simulink model "Schwingerkette_Model"  (R2014b)
settings: Solver=ode45  StartTime=0.0  StopTime=1  RelTol=1e-5
values from neighbouring files (symbols this model uses):
  c = 500    [Schwingerkette_Bearbeitungsfile.m]
  m = 0.5    [Schwingerkette_Bearbeitungsfile.m]
settings Model: Creator=edwardsue  LastModifiedBy=edwardsue

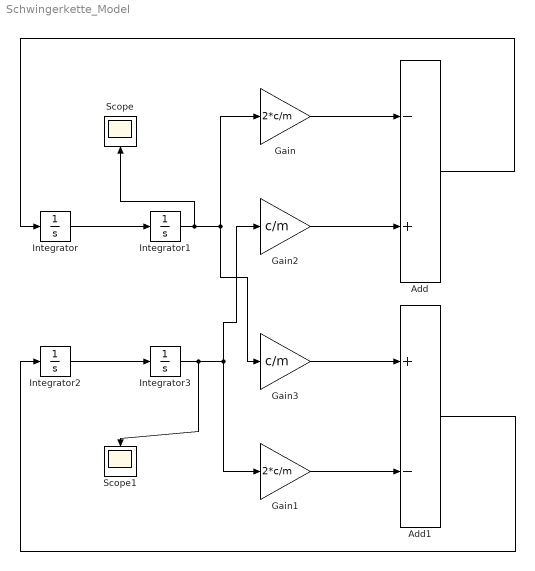
== system Schwingerkette_Model ==
  Add : Sum  Inputs=-+
  Add1 : Sum  Inputs=+-
  Gain : Gain  Gain=2*c/m
  Gain1 : Gain  Gain=2*c/m
  Gain2 : Gain  Gain=c/m
  Gain3 : Gain  Gain=c/m
  Integrator : Integrator
  Integrator1 : Integrator  InitialCondition=0.01
  Integrator2 : Integrator
  Integrator3 : Integrator  InitialCondition=0.01
  Scope : Scope
      settings: YMin=-1  YMax=1.5
  Scope1 : Scope
      settings: YMin=-1  YMax=1.5
  wires:
  Gain/1 -> Add/1
  Gain2/1 -> Add/2
  Integrator/1 -> Integrator1/1
  Integrator1/1 -> Gain3/1, Gain/1, Scope/1
  Integrator2/1 -> Integrator3/1
  Integrator3/1 -> Scope1/1, Gain2/1, Gain1/1
  Add/1 -> Integrator/1
  Gain3/1 -> Add1/1
  Gain1/1 -> Add1/2
  Add1/1 -> Integrator2/1
